simulink model "decentralized_trans"  (R2023b)
settings: Solver=ode45  StartTime=0.0  StopTime=Tf  RelTol=1e-3
undefined symbols (not defined in the file): A_an2, A_an3, Ac_id2, Ac_id3, Ac_mrs2, Ac_mrs3, alpha, b, B_an2, B_an3, Bc_id2, Bc_id3, Bc_mrs2, Bc_mrs3, C2, C3, C_an2, C_an3, C_id2, C_id3, C_opt, Cc_id2, Cc_id3, Cc_mrs2, Cc_mrs3, D_an2, D_an3, Dc_id2, Dc_id3, Dc_mrs2, Dc_mrs3, dx2, dx3, p01, p02, p03, p04, p05, p06, phi02, r_pd1, r_pd2, r_pd3, r_pd4, r_pd5, r_pd6, r_pd_sl1, r_pd_sl2, r_pd_sl3, r_pd_sl4, r_pd_sl5, r_pd_sl6, t1, t2, t3, th, th02, u_max_n1, u_max_n2, u_max_n3 ... (+8)
(part 2 of 2)

== system decentralized_trans/Sixth neighbour/Controller/Controller line follow ==
  uc : Inport
  y : Inport  Port=2
  Ac_id : Gain  Gain=Ac_id2  Multiplication=Matrix(K*u) (u vector)
  Bc_id : Gain  Gain=Bc_id2  Multiplication=Matrix(K*u) (u vector)
  Cc_id : Gain  Gain=Cc_id2  Multiplication=Matrix(K*u) (u vector)
  Dc_id : Gain  Gain=Dc_id2  Multiplication=Matrix(K*u) (u vector)
  Integrator : Integrator  ExternalReset=either  InitialCondition=xc02
  Sum : Sum  Inputs=|++
  Sum1 : Sum  Inputs=++|
  u : Outport
  wires:
  Bc_id/1 -> Sum1/1
  Cc_id/1 -> Sum/1
  uc/1 -> Bc_id/1, Dc_id/1
  Integrator/1 -> Ac_id/1, Cc_id/1
  Dc_id/1 -> Sum/2
  Sum/1 -> u/1
  Ac_id/1 -> Sum1/2
  Sum1/1 -> Integrator/1
  y/1 -> Integrator/2

== system decentralized_trans/Third neighbour/Allocator/Annihilator ==
  v : Inport
  A_an : Gain  Gain=A_an3  Multiplication=Matrix(K*u) (u vector)
  B_an : Gain  Gain=B_an3  Multiplication=Matrix(K*u) (u vector)
  C_an : Gain  Gain=C_an3  Multiplication=Matrix(K*u) (u vector)
  D_an : Gain  Gain=D_an3  Multiplication=Matrix(K*u) (u vector)
  Integrator : Integrator  InitialCondition=xan03
  Sum : Sum  Inputs=|++
  Sum1 : Sum  Inputs=++|
  y_an1 : ToWorkspace  VariableName=yan3  SampleTime=-1
  y_an : Outport
  wires:
  Integrator/1 -> C_an/1, A_an/1
  B_an/1 -> Sum/2
  A_an/1 -> Sum/1
  v/1 -> D_an/1, B_an/1
  Sum/1 -> Integrator/1
  C_an/1 -> Sum1/2
  D_an/1 -> Sum1/1
  Sum1/1 -> y_an1/1, y_an/1

== system decentralized_trans/Third neighbour/Allocator/Optimizer ==
  u : Inport
  u_sat : Inport  Port=2
  C_opt : Gain  Gain=C_opt  Multiplication=Matrix(K*u) (u vector)
  Constant : Constant  Value=alpha
  Dan : Constant  Value=D_an3  VectorParams1D=off
  Integrator : Integrator  InitialCondition=xopt0
  Scope : Scope
  dx_opt : MATLAB Function  TreatAsAtomicUnit=on
  u_max : Constant  Value=u_max_n3
  v : Outport
  wires:
  dx_opt/1(dx_opt) -> Scope/1, Integrator/1
  C_opt/1 -> v/1
  Constant/1 -> dx_opt/1(alpha)
  Dan/1 -> dx_opt/2(D_an)
  u_max/1 -> dx_opt/3(u_max)
  u/1 -> dx_opt/4(u)
  u_sat/1 -> dx_opt/5(u_sat)
  Integrator/1 -> C_opt/1

== system decentralized_trans/Third neighbour/Controller/Controller formation ==
  uc : Inport
  y : Inport  Port=2
  Ac_mrs : Gain  Gain=Ac_mrs3  Multiplication=Matrix(K*u) (u vector)
  Bc_mrs : Gain  Gain=Bc_mrs3  Multiplication=Matrix(K*u) (u vector)
  Cc_mrs : Gain  Gain=Cc_mrs3  Multiplication=Matrix(K*u) (u vector)
  Dc_mrs : Gain  Gain=Dc_mrs3  Multiplication=Matrix(K*u) (u vector)
  Integrator : Integrator  ExternalReset=either  InitialCondition=xc03
  Sum : Sum  Inputs=|++
  Sum1 : Sum  Inputs=++|
  u : Outport
  wires:
  Bc_mrs/1 -> Sum1/1
  Cc_mrs/1 -> Sum/1
  uc/1 -> Bc_mrs/1, Dc_mrs/1
  Integrator/1 -> Ac_mrs/1, Cc_mrs/1
  Dc_mrs/1 -> Sum/2
  Sum/1 -> u/1
  Ac_mrs/1 -> Sum1/2
  Sum1/1 -> Integrator/1
  y/1 -> Integrator/2

== system decentralized_trans/Third neighbour/Controller/Controller line follow ==
  uc : Inport
  y : Inport  Port=2
  Ac_id : Gain  Gain=Ac_id3  Multiplication=Matrix(K*u) (u vector)
  Bc_id : Gain  Gain=Bc_id3  Multiplication=Matrix(K*u) (u vector)
  Cc_id : Gain  Gain=Cc_id3  Multiplication=Matrix(K*u) (u vector)
  Dc_id : Gain  Gain=Dc_id3  Multiplication=Matrix(K*u) (u vector)
  Integrator : Integrator  ExternalReset=either  InitialCondition=xc03
  Sum : Sum  Inputs=|++
  Sum1 : Sum  Inputs=++|
  u : Outport
  wires:
  Bc_id/1 -> Sum1/1
  Cc_id/1 -> Sum/1
  uc/1 -> Bc_id/1, Dc_id/1
  Integrator/1 -> Ac_id/1, Cc_id/1
  Dc_id/1 -> Sum/2
  Sum/1 -> u/1
  Ac_id/1 -> Sum1/2
  Sum1/1 -> Integrator/1
  y/1 -> Integrator/2

== matlab function decentralized_trans/Second neighbour/MRS/MATLAB Function ==
  data: u input; b input; dp output; th input; dth output; phi input; dphi output
function [dp,dth,dphi] = platoon_MRS(u,b,th,phi)

ui = u(3:4);

th1 = th(1);

phi1 = phi(1);

B = eye(2);

Bth = tan(phi1)*[cos(th1) sin(th1)];

Bphi = 1/b*[-sin(th1) cos(th1)];

dp = B*ui;
dth = Bth*ui;
dphi = Bphi*ui;

== matlab function decentralized_trans/Second neighbour/neighbour output/MATLAB Function ==
  data: y1 input; yn output; y2 input; y3 input
function yn = fcn(y1,y2,y3)

yn = [y1;y2;y3];

== matlab function decentralized_trans/Second neighbour/neighbour output/MATLAB Function1 ==
  data: y_lf input; y_MRS output; t input; y_f input; t1 input; t2 input; t3 input
function y_MRS = fcn(y_lf,t,y_f,t1,t2,t3)

%y_MRS = y_f;

if ( t <= t1 )
    y_MRS = y_f;
elseif ( t1 < t && t <= t2 )
    y_MRS = y_lf;
elseif ( t2 < t && t <= t3 )
    y_MRS = y_f;
else
    y_MRS = y_lf;
end

end

== matlab function decentralized_trans/Second neighbour/ref generator/MATLAB Function ==
  data: t input; y output; t1 input; t2 input; t3 input; r_pd input; r_pd2 input; r_line input
function y = switch_ref(t,t1,t2,t3,r_pd,r_pd2,r_line)

y = r_pd;
if ( t <= t1 )
    %disp('one')
    y = r_pd;
end
if ( t1 < t && t <= t2 ) 
    %disp('two')
    y = r_line;
end
if ( t2 < t && t <= t3 )
    %disp('three')
    y = r_pd2;
end
if ( t > t3 )
    %disp('four')
    y = r_line;
end

end

== matlab function decentralized_trans/Second neighbour/ref generator/MATLAB Function1 ==
  data: y output; dx input; state input
function y = fcn(dx,state)

y = state + dx;

end

== matlab function decentralized_trans/Third neighbour/Controller/MATLAB Function ==
  data: u_lf input; yc output; t input; u_f input; t1 input; t2 input; t3 input
function yc = fcn(u_lf,t,u_f, t1,t2,t3)

%yc = u_f;

if ( t <= t1 )
    yc = u_f;
elseif ( t1 < t && t <= t2 )
    yc = u_lf;
elseif ( t2 < t && t <= t3 )
    yc = u_f;
else
    yc = u_lf;
end

end

== matlab function decentralized_trans/Third neighbour/Controller/MATLAB Function1 ==
  data: t input; y output; t1 input; t2 input; t3 input
function y = reset_sig(t,t1,t2,t3)

y = 1;

if ( t1 < t && t <= t2 )
    y = 0;
elseif ( t2 < t && t <= t3 )
    y = 1;
elseif ( t > t3 )
    y = 0;
end

== matlab function decentralized_trans/Third neighbour/MRS/MATLAB Function ==
  data: u input; b input; dp output; th input; dth output; phi input; dphi output
function [dp,dth,dphi] = platoon_MRS(u,b,th,phi)

ui = u(3:4);

th1 = th(1);

phi1 = phi(1);

B = eye(2);

Bth = tan(phi1)*[cos(th1) sin(th1)];

Bphi = 1/b*[-sin(th1) cos(th1)];

dp = B*ui;
dth = Bth*ui;
dphi = Bphi*ui;

== matlab function decentralized_trans/Third neighbour/neighbour output/MATLAB Function ==
  data: y1 input; yn output; y2 input; y3 input
function yn = fcn(y1,y2,y3)

yn = [y1;y2;y3];

== matlab function decentralized_trans/First neighbour/ref generator/MATLAB Function ==
  data: t input; y output; t1 input; t2 input; t3 input; r_pd input; r_pd2 input; r_line input
function y = switch_ref(t,t1,t2,t3,r_pd,r_pd2,r_line)

y = r_pd;
if ( t <= t1 )
    %disp('one')
    y = r_pd;
end
if ( t1 < t && t <= t2 ) 
    %disp('two')
    y = r_line;
end
if ( t2 < t && t <= t3 )
    %disp('three')
    y = r_pd2;
end
if ( t > t3 )
    %disp('four')
    y = r_line;
end

end

== matlab function decentralized_trans/Third neighbour/neighbour output/MATLAB Function1 ==
  data: y_lf input; y_MRS output; t input; y_f input; t1 input; t2 input; t3 input
function y_MRS = fcn(y_lf,t,y_f,t1,t2,t3)

%y_MRS = y_f;

if ( t <= t1 )
    y_MRS = y_f;
elseif ( t1 < t && t <= t2 )
    y_MRS = y_lf;
elseif ( t2 < t && t <= t3 )
    y_MRS = y_f;
else
    y_MRS = y_lf;
end

end

== matlab function decentralized_trans/Third neighbour/ref generator/MATLAB Function ==
  data: t input; y output; t1 input; t2 input; t3 input; r_pd input; r_pd2 input; r_line input
function y = switch_ref(t,t1,t2,t3,r_pd,r_pd2,r_line)

y = r_pd;
if ( t <= t1 )
    %disp('one')
    y = r_pd;
end
if ( t1 < t && t <= t2 ) 
    %disp('two')
    y = r_line;
end
if ( t2 < t && t <= t3 )
    %disp('three')
    y = r_pd2;
end
if ( t > t3 )
    %disp('four')
    y = r_line;
end

end

== matlab function decentralized_trans/Third neighbour/ref generator/MATLAB Function1 ==
  data: y output; dx input; state input
function y = fcn(dx,state)

y = state + dx;

end

== matlab function decentralized_trans/Fourth neighbour/Controller/MATLAB Function ==
  data: u_lf input; yc output; t input; u_f input; t1 input; t2 input; t3 input
function yc = fcn(u_lf,t,u_f, t1,t2,t3)

%yc = u_f;

if ( t <= t1 )
    yc = u_f;
elseif ( t1 < t && t <= t2 )
    yc = u_lf;
elseif ( t2 < t && t <= t3 )
    yc = u_f;
else
    yc = u_lf;
end

end

== matlab function decentralized_trans/Fourth neighbour/Controller/MATLAB Function1 ==
  data: t input; y output; t1 input; t2 input; t3 input
function y = reset_sig(t,t1,t2,t3)

y = 1;

if ( t1 < t && t <= t2 )
    y = 0;
elseif ( t2 < t && t <= t3 )
    y = 1;
elseif ( t > t3 )
    y = 0;
end

== matlab function decentralized_trans/Fourth neighbour/MRS/MATLAB Function ==
  data: u input; b input; dp output; th input; dth output; phi input; dphi output
function [dp,dth,dphi] = platoon_MRS(u,b,th,phi)

ui = u(3:4);

th1 = th(1);

phi1 = phi(1);

B = eye(2);

Bth = tan(phi1)*[cos(th1) sin(th1)];

Bphi = 1/b*[-sin(th1) cos(th1)];

dp = B*ui;
dth = Bth*ui;
dphi = Bphi*ui;

== matlab function decentralized_trans/Fourth neighbour/neighbour output/MATLAB Function ==
  data: y1 input; yn output; y2 input; y3 input
function yn = fcn(y1,y2,y3)

yn = [y1;y2;y3];

== matlab function decentralized_trans/Fourth neighbour/neighbour output/MATLAB Function1 ==
  data: y_lf input; y_MRS output; t input; y_f input; t1 input; t2 input; t3 input
function y_MRS = fcn(y_lf,t,y_f,t1,t2,t3)

%y_MRS = y_f;

if ( t <= t1 )
    y_MRS = y_f;
elseif ( t1 < t && t <= t2 )
    y_MRS = y_lf;
elseif ( t2 < t && t <= t3 )
    y_MRS = y_f;
else
    y_MRS = y_lf;
end

end

== matlab function decentralized_trans/Fourth neighbour/ref generator/MATLAB Function ==
  data: t input; y output; t1 input; t2 input; t3 input; r_pd input; r_pd2 input; r_line input
function y = switch_ref(t,t1,t2,t3,r_pd,r_pd2,r_line)

y = r_pd;
if ( t <= t1 )
    %disp('one')
    y = r_pd;
end
if ( t1 < t && t <= t2 ) 
    %disp('two')
    y = r_line;
end
if ( t2 < t && t <= t3 )
    %disp('three')
    y = r_pd2;
end
if ( t > t3 )
    %disp('four')
    y = r_line;
end

end

== matlab function decentralized_trans/Fourth neighbour/ref generator/MATLAB Function1 ==
  data: y output; dx input; state input
function y = fcn(dx,state)

y = state + dx;

end

== matlab function decentralized_trans/Fifth neighbour/Controller/MATLAB Function ==
  data: u_lf input; yc output; t input; u_f input; t1 input; t2 input; t3 input
function yc = fcn(u_lf,t,u_f, t1,t2,t3)

%yc = u_f;

if ( t <= t1 )
    yc = u_f;
elseif ( t1 < t && t <= t2 )
    yc = u_lf;
elseif ( t2 < t && t <= t3 )
    yc = u_f;
else
    yc = u_lf;
end

end

== matlab function decentralized_trans/Fifth neighbour/Controller/MATLAB Function1 ==
  data: t input; y output; t1 input; t2 input; t3 input
function y = reset_sig(t,t1,t2,t3)

y = 1;

if ( t1 < t && t <= t2 )
    y = 0;
elseif ( t2 < t && t <= t3 )
    y = 1;
elseif ( t > t3 )
    y = 0;
end

== matlab function decentralized_trans/First neighbour/MRS/MATLAB Function ==
  data: u input; b input; dp output; th input; dth output; phi input; dphi output
function [dp,dth,dphi] = platoon_MRS(u,b,th,phi)

ui = u(1:2);

th1 = th(1);

phi1 = phi(1);

B = eye(2);

Bth = tan(phi1)*[cos(th1) sin(th1)];

Bphi = 1/b*[-sin(th1) cos(th1)];

dp = B*ui;
dth = Bth*ui;
dphi = Bphi*ui;

== matlab function decentralized_trans/Fifth neighbour/MRS/MATLAB Function ==
  data: u input; b input; dp output; th input; dth output; phi input; dphi output
function [dp,dth,dphi] = platoon_MRS(u,b,th,phi)

ui = u(3:4);

th1 = th(1);

phi1 = phi(1);

B = eye(2);

Bth = tan(phi1)*[cos(th1) sin(th1)];

Bphi = 1/b*[-sin(th1) cos(th1)];

dp = B*ui;
dth = Bth*ui;
dphi = Bphi*ui;

== matlab function decentralized_trans/Fifth neighbour/neighbour output/MATLAB Function ==
  data: y1 input; yn output; y2 input; y3 input
function yn = fcn(y1,y2,y3)

yn = [y1;y2;y3];

== matlab function decentralized_trans/Fifth neighbour/neighbour output/MATLAB Function1 ==
  data: y_lf input; y_MRS output; t input; y_f input; t1 input; t2 input; t3 input
function y_MRS = fcn(y_lf,t,y_f,t1,t2,t3)

%y_MRS = y_f;

if ( t <= t1 )
    y_MRS = y_f;
elseif ( t1 < t && t <= t2 )
    y_MRS = y_lf;
elseif ( t2 < t && t <= t3 )
    y_MRS = y_f;
else
    y_MRS = y_lf;
end

end

== matlab function decentralized_trans/Fifth neighbour/ref generator/MATLAB Function ==
  data: t input; y output; t1 input; t2 input; t3 input; r_pd input; r_pd2 input; r_line input
function y = switch_ref(t,t1,t2,t3,r_pd,r_pd2,r_line)

y = r_pd;
if ( t <= t1 )
    %disp('one')
    y = r_pd;
end
if ( t1 < t && t <= t2 ) 
    %disp('two')
    y = r_line;
end
if ( t2 < t && t <= t3 )
    %disp('three')
    y = r_pd2;
end
if ( t > t3 )
    %disp('four')
    y = r_line;
end

end

== matlab function decentralized_trans/Fifth neighbour/ref generator/MATLAB Function1 ==
  data: y output; dx input; state input
function y = fcn(dx,state)

y = state + dx;

end

== matlab function decentralized_trans/Sixth neighbour/Controller/MATLAB Function ==
  data: u_lf input; yc output; t input; u_f input; t1 input; t2 input; t3 input
function yc = fcn(u_lf,t,u_f, t1,t2,t3)

%yc = u_f;

if ( t <= t1 )
    yc = u_f;
elseif ( t1 < t && t <= t2 )
    yc = u_lf;
elseif ( t2 < t && t <= t3 )
    yc = u_f;
else
    yc = u_lf;
end

end

== matlab function decentralized_trans/Sixth neighbour/Controller/MATLAB Function1 ==
  data: t input; y output; t1 input; t2 input; t3 input
function y = reset_sig(t,t1,t2,t3)

y = 1;

if ( t1 < t && t <= t2 )
    y = 0;
elseif ( t2 < t && t <= t3 )
    y = 1;
elseif ( t > t3 )
    y = 0;
end

== matlab function decentralized_trans/Sixth neighbour/MRS/MATLAB Function ==
  data: u input; b input; dp output; th input; dth output; phi input; dphi output
function [dp,dth,dphi] = platoon_MRS(u,b,th,phi)

ui = u(3:4);

th1 = th(1);

phi1 = phi(1);

B = eye(2);

Bth = tan(phi1)*[cos(th1) sin(th1)];

Bphi = 1/b*[-sin(th1) cos(th1)];

dp = B*ui;
dth = Bth*ui;
dphi = Bphi*ui;

== matlab function decentralized_trans/Sixth neighbour/neighbour output/MATLAB Function ==
  data: y1 input; yn output; y2 input
function yn = fcn(y1,y2)

yn = [y1;y2];

== matlab function decentralized_trans/Sixth neighbour/neighbour output/MATLAB Function1 ==
  data: y_lf input; y_MRS output; t input; y_f input; t1 input; t2 input; t3 input
function y_MRS = fcn(y_lf,t,y_f,t1,t2,t3)

%y_MRS = y_f;

if ( t <= t1 )
    y_MRS = y_f;
elseif ( t1 < t && t <= t2 )
    y_MRS = y_lf;
elseif ( t2 < t && t <= t3 )
    y_MRS = y_f;
else
    y_MRS = y_lf;
end

end

== matlab function decentralized_trans/Sixth neighbour/ref generator/MATLAB Function ==
  data: t input; y output; t1 input; t2 input; t3 input; r_pd input; r_pd2 input; r_line input
function y = switch_ref(t,t1,t2,t3,r_pd,r_pd2,r_line)

y = r_pd;
if ( t <= t1 )
    %disp('one')
    y = r_pd;
end
if ( t1 < t && t <= t2 ) 
    %disp('two')
    y = r_line;
end
if ( t2 < t && t <= t3 )
    %disp('three')
    y = r_pd2;
end
if ( t > t3 )
    %disp('four')
    y = r_line;
end

end

== matlab function decentralized_trans/First neighbour/ref generator/MATLAB Function1 ==
  data: y output; dx input; state input
function y = fcn(dx,state)

y = state + dx;

end

== matlab function decentralized_trans/Sixth neighbour/ref generator/MATLAB Function1 ==
  data: y output; dx input; state input
function y = fcn(dx,state)

y = state + dx;

end

== matlab function decentralized_trans/First neighbour/neighbour output/MATLAB Function ==
  data: y1 input; yn output; y2 input
function yn = fcn(y1,y2)

yn = [y1;y2];

== matlab function decentralized_trans/First neighbour/Allocator/MATLAB Function ==
  data: e input; G output; th input
function G = fcn(e,th)
norm(e);
eps = th/2;

G=1;

if ( norm(e) < th-eps )
    G = 0;
end
if ( norm(e) > th )
    G = 1;
end
if ( norm(e) <= th && norm(e) >= th-eps )
    G = -2*(norm(e)-(th-eps))^3+3*(norm(e)-(th-eps))^2;
end

== matlab function decentralized_trans/First neighbour/Allocator/Optimizer/dx_opt ==
  data: dx_opt output; alpha input; D_an input; u_max input; u input; u_sat input
function dx_opt = opt_dyn(alpha,D_an,u_max,u,u_sat)

u1_max = u_max(1);
u2_max = u_max(2);
u3_max = u_max(3);
u4_max = u_max(4);

phi = u - u_sat;

par_der = diag([dsat(u(1),u1_max,0.01),dsat(u(2),u2_max,0.01),dsat(u(3),u3_max,0.01),dsat(u(4),u4_max,0.01)]);

grad = phi'*(D_an-par_der*D_an);

dx_opt = -alpha*grad;


% phi = yc+Wan0*x_opt;
% 
% %ss_sat = phi;
% 
% %ss_sat = [u1_max * 2/pi * atan(phi(1));u2_max * 2/pi * atan(phi(2))]; 
% 
% ss_sat = [u1_max * tanh(phi(1));u2_max * tanh(phi(2))]; 
% 
% % if ( abs(phi(1))>=u1_max )
% %     ss_sat(1) = sign(phi(1))*u1_max;
% % end
% % if ( abs(phi(2))>=u2_max )
% %     ss_sat(2) = sign(phi(2))*u2_max;
% % end
% 
% %par_der = diag([(u1_max*2/pi)/(1+(phi(1))^2),(u2_max*2/pi)/(1+(phi(2))^2)]);
% 
% par_der = diag([u1_max/(cosh(phi(1)))^2,u2_max/(cosh(phi(2)))^2]);
% 
% %par_der = diag([dsat(phi(1),u1_max,0.01),dsat(phi(2),u2_max,0.01)]); 
% 
% %grad = (yc+Wan0*x_opt-u_sat)'*(Wan0-par_der*Wan0);
% 
% grad = (yc+Wan0*x_opt-ss_sat)'*(Wan0-par_der*Wan0);
% 
% dx_opt = -alpha*grad;

== matlab function decentralized_trans/Sixth neighbour/Allocator/MATLAB Function ==
  data: e input; G output; th input
function G = fcn(e,th)
norm(e);
eps = th/2;

G=1;

if ( norm(e) < th-eps )
    G = 0;
end
if ( norm(e) > th )
    G = 1;
end
if ( norm(e) <= th && norm(e) >= th-eps )
    G = -2*(norm(e)-(th-eps))^3+3*(norm(e)-(th-eps))^2;
end

== matlab function decentralized_trans/Sixth neighbour/Allocator/Optimizer/dx_opt ==
  data: dx_opt output; alpha input; D_an input; u_max input; u input; u_sat input
function dx_opt = opt_dyn(alpha,D_an,u_max,u,u_sat)

u1_max = u_max(1);
u2_max = u_max(2);
u3_max = u_max(3);
u4_max = u_max(4);

phi = u - u_sat;

par_der = diag([dsat(u(1),u1_max,0.01),dsat(u(2),u2_max,0.01),dsat(u(3),u3_max,0.01),dsat(u(4),u4_max,0.01)]);

grad = phi'*(D_an-par_der*D_an);

dx_opt = -alpha*grad;


% phi = yc+Wan0*x_opt;
% 
% %ss_sat = phi;
% 
% %ss_sat = [u1_max * 2/pi * atan(phi(1));u2_max * 2/pi * atan(phi(2))]; 
% 
% ss_sat = [u1_max * tanh(phi(1));u2_max * tanh(phi(2))]; 
% 
% % if ( abs(phi(1))>=u1_max )
% %     ss_sat(1) = sign(phi(1))*u1_max;
% % end
% % if ( abs(phi(2))>=u2_max )
% %     ss_sat(2) = sign(phi(2))*u2_max;
% % end
% 
% %par_der = diag([(u1_max*2/pi)/(1+(phi(1))^2),(u2_max*2/pi)/(1+(phi(2))^2)]);
% 
% par_der = diag([u1_max/(cosh(phi(1)))^2,u2_max/(cosh(phi(2)))^2]);
% 
% %par_der = diag([dsat(phi(1),u1_max,0.01),dsat(phi(2),u2_max,0.01)]); 
% 
% %grad = (yc+Wan0*x_opt-u_sat)'*(Wan0-par_der*Wan0);
% 
% grad = (yc+Wan0*x_opt-ss_sat)'*(Wan0-par_der*Wan0);
% 
% dx_opt = -alpha*grad;

== matlab function decentralized_trans/Second neighbour/Allocator/MATLAB Function ==
  data: e input; G output; th input
function G = fcn(e,th)
norm(e);
eps = th/2;

G=1;

if ( norm(e) < th-eps )
    G = 0;
end
if ( norm(e) > th )
    G = 1;
end
if ( norm(e) <= th && norm(e) >= th-eps )
    G = -2*(norm(e)-(th-eps))^3+3*(norm(e)-(th-eps))^2;
end

== matlab function decentralized_trans/Second neighbour/Allocator/Optimizer/dx_opt ==
  data: dx_opt output; alpha input; D_an input; u_max input; u input; u_sat input
function dx_opt = opt_dyn(alpha,D_an,u_max,u,u_sat)

u1_max = u_max(1);
u2_max = u_max(2);
u3_max = u_max(3);
u4_max = u_max(4);
u5_max = u_max(5);
u6_max = u_max(6);

phi = u - u_sat;

par_der = diag([dsat(u(1),u1_max,0.01),dsat(u(2),u2_max,0.01),dsat(u(3),u3_max,0.01),dsat(u(4),u4_max,0.01),dsat(u(5),u5_max,0.01),dsat(u(6),u6_max,0.01)]);

grad = phi'*(D_an-par_der*D_an);

dx_opt = -alpha*grad;


% phi = yc+Wan0*x_opt;
% 
% %ss_sat = phi;
% 
% %ss_sat = [u1_max * 2/pi * atan(phi(1));u2_max * 2/pi * atan(phi(2))]; 
% 
% ss_sat = [u1_max * tanh(phi(1));u2_max * tanh(phi(2))]; 
% 
% % if ( abs(phi(1))>=u1_max )
% %     ss_sat(1) = sign(phi(1))*u1_max;
% % end
% % if ( abs(phi(2))>=u2_max )
% %     ss_sat(2) = sign(phi(2))*u2_max;
% % end
% 
% %par_der = diag([(u1_max*2/pi)/(1+(phi(1))^2),(u2_max*2/pi)/(1+(phi(2))^2)]);
% 
% par_der = diag([u1_max/(cosh(phi(1)))^2,u2_max/(cosh(phi(2)))^2]);
% 
% %par_der = diag([dsat(phi(1),u1_max,0.01),dsat(phi(2),u2_max,0.01)]); 
% 
% %grad = (yc+Wan0*x_opt-u_sat)'*(Wan0-par_der*Wan0);
% 
% grad = (yc+Wan0*x_opt-ss_sat)'*(Wan0-par_der*Wan0);
% 
% dx_opt = -alpha*grad;

== matlab function decentralized_trans/First neighbour/Controller/MATLAB Function ==
  data: u_lf input; yc output; t input; u_f input; t1 input; t2 input; t3 input
function yc = fcn(u_lf,t,u_f, t1,t2,t3)

%yc = u_f;

if ( t <= t1 )
    yc = u_f;
elseif ( t1 < t && t <= t2 )
    yc = u_lf;
elseif ( t2 < t && t <= t3 )
    yc = u_f;
else
    yc = u_lf;
end

end

== matlab function decentralized_trans/Third neighbour/Allocator/MATLAB Function ==
  data: e input; G output; th input
function G = fcn(e,th)
norm(e);
eps = th/2;

G=1;

if ( norm(e) < th-eps )
    G = 0;
end
if ( norm(e) > th )
    G = 1;
end
if ( norm(e) <= th && norm(e) >= th-eps )
    G = -2*(norm(e)-(th-eps))^3+3*(norm(e)-(th-eps))^2;
end

== matlab function decentralized_trans/Third neighbour/Allocator/Optimizer/dx_opt ==
  data: dx_opt output; alpha input; D_an input; u_max input; u input; u_sat input
function dx_opt = opt_dyn(alpha,D_an,u_max,u,u_sat)

u1_max = u_max(1);
u2_max = u_max(2);
u3_max = u_max(3);
u4_max = u_max(4);
u5_max = u_max(5);
u6_max = u_max(6);

phi = u - u_sat;

par_der = diag([dsat(u(1),u1_max,0.01),dsat(u(2),u2_max,0.01),dsat(u(3),u3_max,0.01),dsat(u(4),u4_max,0.01),dsat(u(5),u5_max,0.01),dsat(u(6),u6_max,0.01)]);

grad = phi'*(D_an-par_der*D_an);

dx_opt = -alpha*grad;


% phi = yc+Wan0*x_opt;
% 
% %ss_sat = phi;
% 
% %ss_sat = [u1_max * 2/pi * atan(phi(1));u2_max * 2/pi * atan(phi(2))]; 
% 
% ss_sat = [u1_max * tanh(phi(1));u2_max * tanh(phi(2))]; 
% 
% % if ( abs(phi(1))>=u1_max )
% %     ss_sat(1) = sign(phi(1))*u1_max;
% % end
% % if ( abs(phi(2))>=u2_max )
% %     ss_sat(2) = sign(phi(2))*u2_max;
% % end
% 
% %par_der = diag([(u1_max*2/pi)/(1+(phi(1))^2),(u2_max*2/pi)/(1+(phi(2))^2)]);
% 
% par_der = diag([u1_max/(cosh(phi(1)))^2,u2_max/(cosh(phi(2)))^2]);
% 
% %par_der = diag([dsat(phi(1),u1_max,0.01),dsat(phi(2),u2_max,0.01)]); 
% 
% %grad = (yc+Wan0*x_opt-u_sat)'*(Wan0-par_der*Wan0);
% 
% grad = (yc+Wan0*x_opt-ss_sat)'*(Wan0-par_der*Wan0);
% 
% dx_opt = -alpha*grad;

== matlab function decentralized_trans/Fourth neighbour/Allocator/MATLAB Function ==
  data: e input; G output; th input
function G = fcn(e,th)
norm(e);
eps = th/2;

G=1;

if ( norm(e) < th-eps )
    G = 0;
end
if ( norm(e) > th )
    G = 1;
end
if ( norm(e) <= th && norm(e) >= th-eps )
    G = -2*(norm(e)-(th-eps))^3+3*(norm(e)-(th-eps))^2;
end

== matlab function decentralized_trans/Fourth neighbour/Allocator/Optimizer/dx_opt ==
  data: dx_opt output; alpha input; D_an input; u_max input; u input; u_sat input
function dx_opt = opt_dyn(alpha,D_an,u_max,u,u_sat)

u1_max = u_max(1);
u2_max = u_max(2);
u3_max = u_max(3);
u4_max = u_max(4);
u5_max = u_max(5);
u6_max = u_max(6);

phi = u - u_sat;

par_der = diag([dsat(u(1),u1_max,0.01),dsat(u(2),u2_max,0.01),dsat(u(3),u3_max,0.01),dsat(u(4),u4_max,0.01),dsat(u(5),u5_max,0.01),dsat(u(6),u6_max,0.01)]);

grad = phi'*(D_an-par_der*D_an);

dx_opt = -alpha*grad;


% phi = yc+Wan0*x_opt;
% 
% %ss_sat = phi;
% 
% %ss_sat = [u1_max * 2/pi * atan(phi(1));u2_max * 2/pi * atan(phi(2))]; 
% 
% ss_sat = [u1_max * tanh(phi(1));u2_max * tanh(phi(2))]; 
% 
% % if ( abs(phi(1))>=u1_max )
% %     ss_sat(1) = sign(phi(1))*u1_max;
% % end
% % if ( abs(phi(2))>=u2_max )
% %     ss_sat(2) = sign(phi(2))*u2_max;
% % end
% 
% %par_der = diag([(u1_max*2/pi)/(1+(phi(1))^2),(u2_max*2/pi)/(1+(phi(2))^2)]);
% 
% par_der = diag([u1_max/(cosh(phi(1)))^2,u2_max/(cosh(phi(2)))^2]);
% 
% %par_der = diag([dsat(phi(1),u1_max,0.01),dsat(phi(2),u2_max,0.01)]); 
% 
% %grad = (yc+Wan0*x_opt-u_sat)'*(Wan0-par_der*Wan0);
% 
% grad = (yc+Wan0*x_opt-ss_sat)'*(Wan0-par_der*Wan0);
% 
% dx_opt = -alpha*grad;

== matlab function decentralized_trans/Fifth neighbour/Allocator/MATLAB Function ==
  data: e input; G output; th input
function G = fcn(e,th)
norm(e);
eps = th/2;

G=1;

if ( norm(e) < th-eps )
    G = 0;
end
if ( norm(e) > th )
    G = 1;
end
if ( norm(e) <= th && norm(e) >= th-eps )
    G = -2*(norm(e)-(th-eps))^3+3*(norm(e)-(th-eps))^2;
end

== matlab function decentralized_trans/Fifth neighbour/Allocator/Optimizer/dx_opt ==
  data: dx_opt output; alpha input; D_an input; u_max input; u input; u_sat input
function dx_opt = opt_dyn(alpha,D_an,u_max,u,u_sat)

u1_max = u_max(1);
u2_max = u_max(2);
u3_max = u_max(3);
u4_max = u_max(4);
u5_max = u_max(5);
u6_max = u_max(6);

phi = u - u_sat;

par_der = diag([dsat(u(1),u1_max,0.01),dsat(u(2),u2_max,0.01),dsat(u(3),u3_max,0.01),dsat(u(4),u4_max,0.01),dsat(u(5),u5_max,0.01),dsat(u(6),u6_max,0.01)]);

grad = phi'*(D_an-par_der*D_an);

dx_opt = -alpha*grad;


% phi = yc+Wan0*x_opt;
% 
% %ss_sat = phi;
% 
% %ss_sat = [u1_max * 2/pi * atan(phi(1));u2_max * 2/pi * atan(phi(2))]; 
% 
% ss_sat = [u1_max * tanh(phi(1));u2_max * tanh(phi(2))]; 
% 
% % if ( abs(phi(1))>=u1_max )
% %     ss_sat(1) = sign(phi(1))*u1_max;
% % end
% % if ( abs(phi(2))>=u2_max )
% %     ss_sat(2) = sign(phi(2))*u2_max;
% % end
% 
% %par_der = diag([(u1_max*2/pi)/(1+(phi(1))^2),(u2_max*2/pi)/(1+(phi(2))^2)]);
% 
% par_der = diag([u1_max/(cosh(phi(1)))^2,u2_max/(cosh(phi(2)))^2]);
% 
% %par_der = diag([dsat(phi(1),u1_max,0.01),dsat(phi(2),u2_max,0.01)]); 
% 
% %grad = (yc+Wan0*x_opt-u_sat)'*(Wan0-par_der*Wan0);
% 
% grad = (yc+Wan0*x_opt-ss_sat)'*(Wan0-par_der*Wan0);
% 
% dx_opt = -alpha*grad;

== matlab function decentralized_trans/First neighbour/neighbour output/MATLAB Function1 ==
  data: y_lf input; y_MRS output; t input; y_f input; t1 input; t2 input; t3 input
function y_MRS = fcn(y_lf,t,y_f,t1,t2,t3)

%y_MRS = y_f;

if ( t <= t1 )
    y_MRS = y_f;
elseif ( t1 < t && t <= t2 )
    y_MRS = y_lf;
elseif ( t2 < t && t <= t3 )
    y_MRS = y_f;
else
    y_MRS = y_lf;
end

end

== matlab function decentralized_trans/First neighbour/Controller/MATLAB Function1 ==
  data: t input; y output; t1 input; t2 input; t3 input
function y = reset_sig(t,t1,t2,t3)

y = 1;

if ( t1 < t && t <= t2 )
    y = 0;
elseif ( t2 < t && t <= t3 )
    y = 1;
elseif ( t > t3 )
    y = 0;
end

== matlab function decentralized_trans/Second neighbour/Controller/MATLAB Function ==
  data: u_lf input; yc output; t input; u_f input; t1 input; t2 input; t3 input
function yc = fcn(u_lf,t,u_f, t1,t2,t3)

%yc = u_f;

if ( t <= t1 )
    yc = u_f;
elseif ( t1 < t && t <= t2 )
    yc = u_lf;
elseif ( t2 < t && t <= t3 )
    yc = u_f;
else
    yc = u_lf;
end

end

== matlab function decentralized_trans/Second neighbour/Controller/MATLAB Function1 ==
  data: t input; y output; t1 input; t2 input; t3 input
function y = reset_sig(t,t1,t2,t3)

y = 1;

if ( t1 < t && t <= t2 )
    y = 0;
elseif ( t2 < t && t <= t3 )
    y = 1;
elseif ( t > t3 )
    y = 0;
end
